simulink model "prova_simulink"  (R2021a)
settings: Solver=VariableStepAuto  StartTime=0.0  StopTime=10.0  RelTol=1e-3
undefined symbols (not defined in the file): C, epsilon1, epsilon2, nre, nse, polo, R_d, RR_s, ue
libraries: cstblocks x5
settings Model: Creator=lucia  LastModifiedBy=lucia

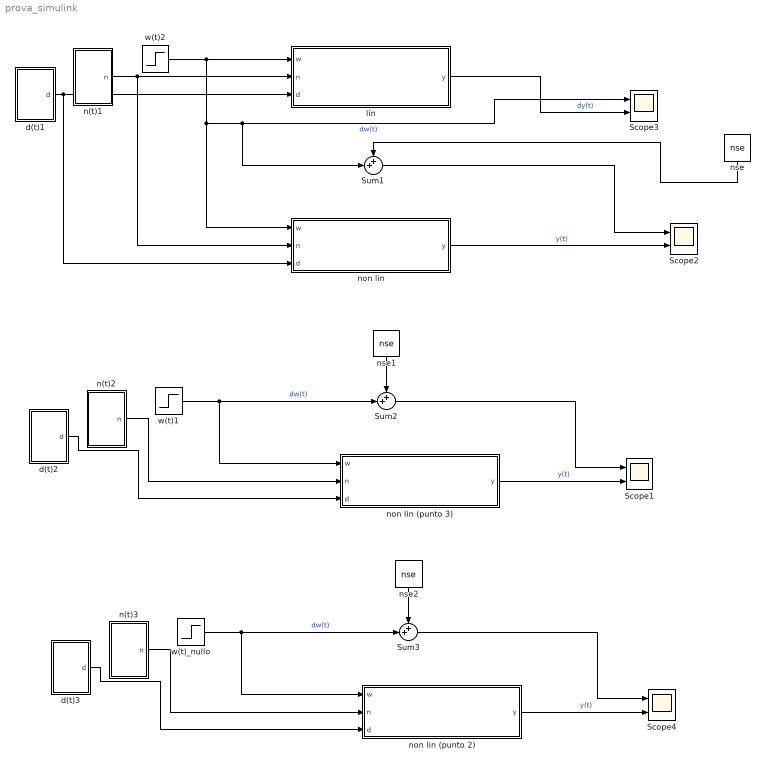
== system prova_simulink ==
  Scope{1..4} (4 alike) : Scope  NumInputPorts=2
  Sum1 : Sum  Inputs=++|
  Sum2 : Sum  Inputs=++|
  Sum3 : Sum  Inputs=++|
  d(t)1 : Subsystem
  d(t)2 : Subsystem
  d(t)3 : Subsystem
  lin : Subsystem
  n(t)1 : Subsystem
  n(t)2 : Subsystem
  n(t)3 : Subsystem
  non lin : Subsystem
  non lin (punto 2) : Subsystem
  non lin (punto 3) : Subsystem
  nse : Constant  Value=nse
  nse1 : Constant  Value=nse
  nse2 : Constant  Value=nse
  w(t)1 : Step  Time=0  After=0  SampleTime=0
  w(t)2 : Step  Time=0  After=-25  SampleTime=0
  w(t)_nullo : Step  Time=0  After=0  SampleTime=0
  wires:
  lin/1(y) -> Scope3/2  "dy(t)"
  d(t)1/1(d) -> non lin/3(d), lin/3(d)
  n(t)1/1(n) -> non lin/2(n), lin/2(n)
  w(t)2/1 -> Sum1/2, Scope3/1, non lin/1(w), lin/1(w)  "dw(t)"
  non lin/1(y) -> Scope2/2  "y(t)"
  Sum1/1 -> Scope2/1
  nse/1 -> Sum1/1
  Sum2/1 -> Scope1/1
  d(t)2/1(d) -> non lin (punto 3)/3(d)
  w(t)1/1 -> non lin (punto 3)/1(w), Sum2/2  "dw(t)"
  nse1/1 -> Sum2/1
  n(t)2/1(n) -> non lin (punto 3)/2(n)
  non lin (punto 3)/1(y) -> Scope1/2  "y(t)"
  nse2/1 -> Sum3/1
  n(t)3/1(n) -> non lin (punto 2)/2(n)
  w(t)_nullo/1 -> non lin (punto 2)/1(w), Sum3/2  "dw(t)"
  non lin (punto 2)/1(y) -> Scope4/2  "y(t)"
  d(t)3/1(d) -> non lin (punto 2)/3(d)
  Sum3/1 -> Scope4/1

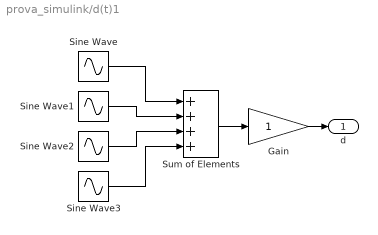
== system prova_simulink/d(t)1 ==
  Gain : Gain
  Sine Wave : Sin  Amplitude=8  Frequency=0.0375  SampleTime=0
  Sine Wave1 : Sin  Amplitude=8  Frequency=0.0375*2  SampleTime=0
  Sine Wave2 : Sin  Amplitude=8  Frequency=0.0375*3  SampleTime=0
  Sine Wave3 : Sin  Amplitude=8  Frequency=0.0375*4  SampleTime=0
  Sum of Elements : Sum  Inputs=++++  InputSameDT=on
  d : Outport
  wires:
  Sum of Elements/1 -> Gain/1
  Sine Wave2/1 -> Sum of Elements/3
  Gain/1 -> d/1
  Sine Wave/1 -> Sum of Elements/1
  Sine Wave3/1 -> Sum of Elements/4
  Sine Wave1/1 -> Sum of Elements/2

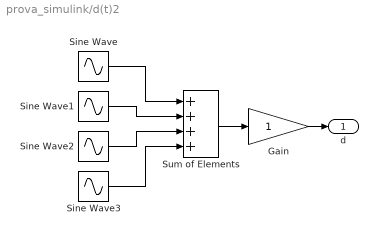
== system prova_simulink/d(t)2 ==
  Gain : Gain
  Sine Wave : Sin  Amplitude=8  Frequency=0.0375  SampleTime=0
  Sine Wave1 : Sin  Amplitude=8  Frequency=0.0375*2  SampleTime=0
  Sine Wave2 : Sin  Amplitude=8  Frequency=0.0375*3  SampleTime=0
  Sine Wave3 : Sin  Amplitude=8  Frequency=0.0375*4  SampleTime=0
  Sum of Elements : Sum  Inputs=++++  InputSameDT=on
  d : Outport
  wires:
  Sum of Elements/1 -> Gain/1
  Sine Wave2/1 -> Sum of Elements/3
  Gain/1 -> d/1
  Sine Wave/1 -> Sum of Elements/1
  Sine Wave3/1 -> Sum of Elements/4
  Sine Wave1/1 -> Sum of Elements/2

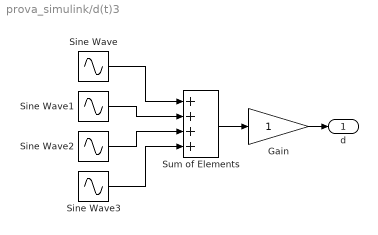
== system prova_simulink/d(t)3 ==
  Gain : Gain
  Sine Wave : Sin  Amplitude=8  Frequency=0.0375  SampleTime=0
  Sine Wave1 : Sin  Amplitude=8  Frequency=0.0375*2  SampleTime=0
  Sine Wave2 : Sin  Amplitude=8  Frequency=0.0375*3  SampleTime=0
  Sine Wave3 : Sin  Amplitude=8  Frequency=0.0375*4  SampleTime=0
  Sum of Elements : Sum  Inputs=++++  InputSameDT=on
  d : Outport
  wires:
  Sum of Elements/1 -> Gain/1
  Sine Wave2/1 -> Sum of Elements/3
  Gain/1 -> d/1
  Sine Wave/1 -> Sum of Elements/1
  Sine Wave3/1 -> Sum of Elements/4
  Sine Wave1/1 -> Sum of Elements/2

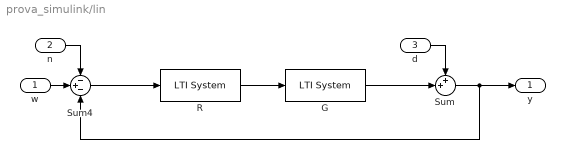
== system prova_simulink/lin ==
  w : Inport
  n : Inport  Port=2
  d : Inport  Port=3
  G : cstblocks/LTI System  sys=GG  IC=[]
  R : cstblocks/LTI System  sys=R_d*RR_s*polo  IC=[]
  Sum : Sum  Inputs=++|
  Sum4 : Sum  Inputs=-+-
  y : Outport
  wires:
  w/1 -> Sum4/2
  n/1 -> Sum4/1
  Sum/1 -> y/1, Sum4/3
  d/1 -> Sum/1
  Sum4/1 -> R/1
  R/1 -> G/1
  G/1 -> Sum/2

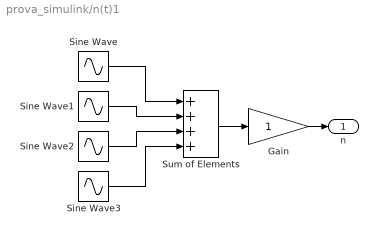
== system prova_simulink/n(t)1 ==
  Gain : Gain
  Sine Wave : Sin  Amplitude=5  Frequency=3.5e3  SampleTime=0
  Sine Wave1 : Sin  Amplitude=5  Frequency=2*3.5e3  SampleTime=0
  Sine Wave2 : Sin  Amplitude=5  Frequency=3*3.5e3  SampleTime=0
  Sine Wave3 : Sin  Amplitude=5  Frequency=4*3.5e3  SampleTime=0
  Sum of Elements : Sum  Inputs=++++  InputSameDT=on
  n : Outport
  wires:
  Sum of Elements/1 -> Gain/1
  Sine Wave2/1 -> Sum of Elements/3
  Gain/1 -> n/1
  Sine Wave/1 -> Sum of Elements/1
  Sine Wave3/1 -> Sum of Elements/4
  Sine Wave1/1 -> Sum of Elements/2

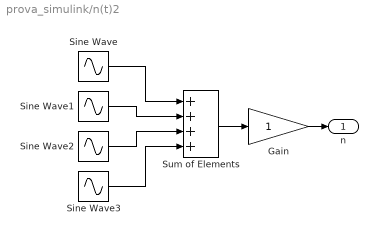
== system prova_simulink/n(t)2 ==
  Gain : Gain
  Sine Wave : Sin  Amplitude=5  Frequency=3.5e3  SampleTime=0
  Sine Wave1 : Sin  Amplitude=5  Frequency=2*3.5e3  SampleTime=0
  Sine Wave2 : Sin  Amplitude=5  Frequency=3*3.5e3  SampleTime=0
  Sine Wave3 : Sin  Amplitude=5  Frequency=4*3.5e3  SampleTime=0
  Sum of Elements : Sum  Inputs=++++  InputSameDT=on
  n : Outport
  wires:
  Sum of Elements/1 -> Gain/1
  Sine Wave2/1 -> Sum of Elements/3
  Gain/1 -> n/1
  Sine Wave/1 -> Sum of Elements/1
  Sine Wave3/1 -> Sum of Elements/4
  Sine Wave1/1 -> Sum of Elements/2

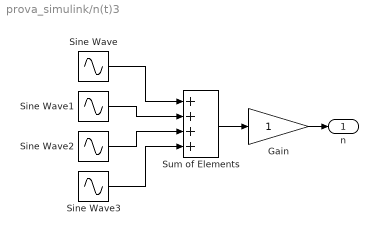
== system prova_simulink/n(t)3 ==
  Gain : Gain
  Sine Wave : Sin  Amplitude=5  Frequency=3.5e3  SampleTime=0
  Sine Wave1 : Sin  Amplitude=5  Frequency=2*3.5e3  SampleTime=0
  Sine Wave2 : Sin  Amplitude=5  Frequency=3*3.5e3  SampleTime=0
  Sine Wave3 : Sin  Amplitude=5  Frequency=4*3.5e3  SampleTime=0
  Sum of Elements : Sum  Inputs=++++  InputSameDT=on
  n : Outport
  wires:
  Sum of Elements/1 -> Gain/1
  Sine Wave2/1 -> Sum of Elements/3
  Gain/1 -> n/1
  Sine Wave/1 -> Sum of Elements/1
  Sine Wave3/1 -> Sum of Elements/4
  Sine Wave1/1 -> Sum of Elements/2

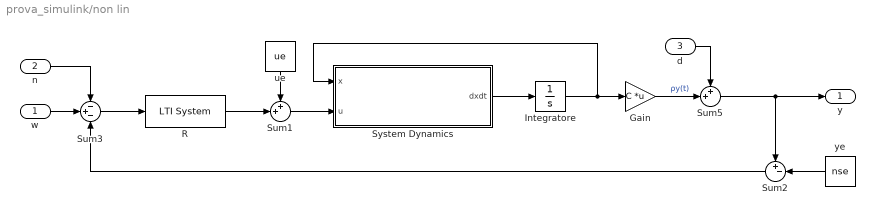
== system prova_simulink/non lin ==
  w : Inport
  n : Inport  Port=2
  d : Inport  Port=3
  Gain : Gain  Gain=C  Multiplication=Matrix(K*u)
  Integratore : Integrator  InitialCondition=[nse, nre]
  R : cstblocks/LTI System  sys=R_d*RR_s*polo  IC=[]
  Sum1 : Sum  Inputs=++|
  Sum2 : Sum  Inputs=+-|
  Sum3 : Sum  Inputs=-+-
  Sum5 : Sum  Inputs=++|
  System Dynamics : MATLAB Function  TreatAsAtomicUnit=on
  ue : Constant  Value=ue
  ye : Constant  Value=nse
  y : Outport
  wires:
  Integratore/1 -> System Dynamics/1(x), Gain/1
  ye/1 -> Sum2/2
  Sum2/1 -> Sum3/3
  Sum5/1 -> y/1, Sum2/1
  Sum1/1 -> System Dynamics/2(u)
  System Dynamics/1(dxdt) -> Integratore/1
  ue/1 -> Sum1/1
  n/1 -> Sum3/1
  Gain/1 -> Sum5/2  "ρy(t)"
  d/1 -> Sum5/1
  w/1 -> Sum3/2
  Sum3/1 -> R/1
  R/1 -> Sum1/2

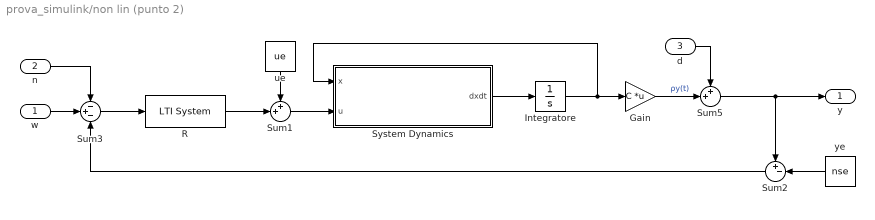
== system prova_simulink/non lin (punto 2) ==
  w : Inport
  n : Inport  Port=2
  d : Inport  Port=3
  Gain : Gain  Gain=C  Multiplication=Matrix(K*u)
  Integratore : Integrator  InitialCondition=[nse*(1+epsilon1), nre*(1+epsilon2)]
  R : cstblocks/LTI System  sys=R_d*RR_s*polo  IC=[]
  Sum1 : Sum  Inputs=++|
  Sum2 : Sum  Inputs=+-|
  Sum3 : Sum  Inputs=-+-
  Sum5 : Sum  Inputs=++|
  System Dynamics : MATLAB Function  TreatAsAtomicUnit=on
  ue : Constant  Value=ue
  ye : Constant  Value=nse
  y : Outport
  wires:
  Integratore/1 -> System Dynamics/1(x), Gain/1
  ye/1 -> Sum2/2
  Sum2/1 -> Sum3/3
  Sum5/1 -> y/1, Sum2/1
  Sum1/1 -> System Dynamics/2(u)
  System Dynamics/1(dxdt) -> Integratore/1
  ue/1 -> Sum1/1
  n/1 -> Sum3/1
  Gain/1 -> Sum5/2  "ρy(t)"
  d/1 -> Sum5/1
  w/1 -> Sum3/2
  Sum3/1 -> R/1
  R/1 -> Sum1/2

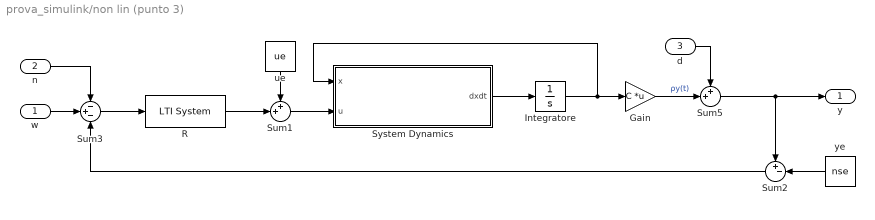
== system prova_simulink/non lin (punto 3) ==
  w : Inport
  n : Inport  Port=2
  d : Inport  Port=3
  Gain : Gain  Gain=C  Multiplication=Matrix(K*u)
  Integratore : Integrator  InitialCondition=[nse, nre]
  R : cstblocks/LTI System  sys=R_d*RR_s*polo  IC=[]
  Sum1 : Sum  Inputs=++|
  Sum2 : Sum  Inputs=+-|
  Sum3 : Sum  Inputs=-+-
  Sum5 : Sum  Inputs=++|
  System Dynamics : MATLAB Function  TreatAsAtomicUnit=on
  ue : Constant  Value=ue
  ye : Constant  Value=nse
  y : Outport
  wires:
  Integratore/1 -> System Dynamics/1(x), Gain/1
  ye/1 -> Sum2/2
  Sum2/1 -> Sum3/3
  Sum5/1 -> y/1, Sum2/1
  Sum1/1 -> System Dynamics/2(u)
  System Dynamics/1(dxdt) -> Integratore/1
  ue/1 -> Sum1/1
  n/1 -> Sum3/1
  Gain/1 -> Sum5/2  "ρy(t)"
  d/1 -> Sum5/1
  w/1 -> Sum3/2
  Sum3/1 -> R/1
  R/1 -> Sum1/2

== matlab function prova_simulink/non lin (punto 3)/System Dynamics ==
  data: x input; u input; dxdt output


function dxdt = systemDynamics(x,u)


beta = 0.1;
alfa = 0.2;
rs=1.6;
rr=1.6;
ms=0.75;
mr=0.1;
gamma=0.05;
K=900;
%nse=300;
%nre=600;
%ue=0;


% bisogna capire da cosa è composta l'uscita per verdere l'ordine
ns=x(1);
nr=x(2);
cf=u;

dnsdt=rs*(1-(ns+nr)/K)*ns-ms*cf*ns-beta*ns+gamma*nr-alfa*cf*ns;
dnrdt=rr*(1-(ns+nr)/K)*nr-mr*cf*nr+beta*ns-gamma*nr+alfa*cf*ns;
dxdt = [dnsdt; dnrdt;];

== matlab function prova_simulink/non lin (punto 2)/System Dynamics ==
  data: x input; u input; dxdt output


function dxdt = systemDynamics(x,u)


beta = 0.1;
alfa = 0.2;
rs=1.6;
rr=1.6;
ms=0.75;
mr=0.1;
gamma=0.05;
K=900;
%nse=300;
%nre=600;
%ue=0;


% bisogna capire da cosa è composta l'uscita per verdere l'ordine
ns=x(1);
nr=x(2);
cf=u;

dnsdt=rs*(1-(ns+nr)/K)*ns-ms*cf*ns-beta*ns+gamma*nr-alfa*cf*ns;
dnrdt=rr*(1-(ns+nr)/K)*nr-mr*cf*nr+beta*ns-gamma*nr+alfa*cf*ns;
dxdt = [dnsdt; dnrdt;];

== matlab function prova_simulink/non lin/System Dynamics ==
  data: x input; u input; dxdt output


function dxdt = systemDynamics(x,u)


beta = 0.1;
alfa = 0.2;
rs=1.6;
rr=1.6;
ms=0.75;
mr=0.1;
gamma=0.05;
K=900;
%nse=300;
%nre=600;
%ue=0;


% bisogna capire da cosa è composta l'uscita per verdere l'ordine
ns=x(1);
nr=x(2);
cf=u;

dnsdt=rs*(1-(ns+nr)/K)*ns-ms*cf*ns-beta*ns+gamma*nr-alfa*cf*ns;
dnrdt=rr*(1-(ns+nr)/K)*nr-mr*cf*nr+beta*ns-gamma*nr+alfa*cf*ns;
dxdt = [dnsdt; dnrdt;];
